simulink model "matrix"  (R2023a)
settings: Solver=VariableStepAuto  StartTime=0.0  StopTime=1  RelTol=1e-3
libraries: spsDiodeLib x8, spsIGBTLib x8, spsVoltageMeasurementLib x2, spsACVoltageSourceLib x1, sps_lib x1, spsSeriesRLCBranchLib x1
settings Model: Creator=burra  LastModifiedBy=vande

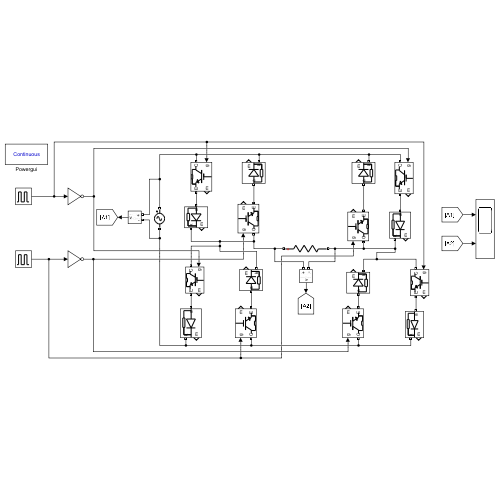
[thumbnail: Simulink's stored preview of the top-level diagram]
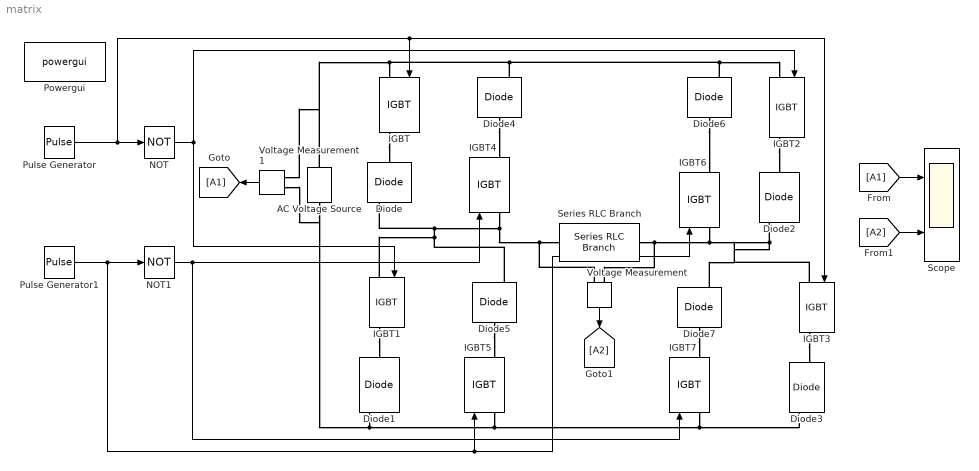
== system matrix ==
  AC Voltage Source : spsACVoltageSourceLib/AC Voltage Source  Amplitude=230  Phase=0  Frequency=50  SampleTime=0  Measurements=None  BusType=swing  Pref=10e3  Qref=0  Qmin=-inf  Qmax=+inf
  Diode{,1..7} (8 alike) : spsDiodeLib/Diode  Ron=0.001  Lon=0  Vf=0.8  IC=0  UseSnubber=0  Rs=500  Cs=250e-9  Measurements=on
  IGBT{,1..7} (8 alike) : spsIGBTLib/IGBT  Ron=0.001  Lon=0  Vf=1  Tf=1e-6  Tt=2e-6  IC=0  Rs=1e5  Cs=inf  Measurements=on
  NOT : Logic  Operator=NOT  IconShape=distinctive  AllPortsSameDT=off  OutDataTypeStr=boolean
  NOT1 : Logic  Operator=NOT  IconShape=distinctive  AllPortsSameDT=off  OutDataTypeStr=boolean
  Powergui : sps_lib/powergui  Priority=1  SimulationMode=Continuous  SampleTime=50e-6  frequency=60  Iterations=50  frequencyindice=50  Pbase=100e6  ErrMax=1e-4  UnitsV=kV  UnitsW=MW  buscounter=0  FunctionMessages=off  echomessages=off  EnableUseOfTLC=off  CurrentSourceSwitches=off  DisableSnubberDevices=off  DisableRonSwitches=off  DisableVfSwitches=off  DisplayEquations=off  AutomaticDiscreteSolvers=off  SolverType=Tustin/Backward Euler (TBE)  Interpol=off  ExternalGateDelay=off  methode=off  Ts=100  x0status=blocks  SPID=on  SwTol=0  HookPort=off  NonlinearTolerance=1e-4  nMaxIteration=100  ContinueOnMaxIteration=off  RestoreLinks=warning  ResistiveCurrentMeasurement=off  Frange=[0:2:500]  Ylog=off  Xlog=on  ShowGrid=off  save=off  variable=ZData  structure=0  ZoomFFT=off  StartTime=0.0  cycles=1  DisplayStyle=1  fundamental=60  FreqAxis=off  MaxFrequency=1000  frequencyindicesteady=1  RmsSteady=1  display=off
  Pulse Generator : DiscretePulseGenerator  PulseType=Time based  Period=0.001  PulseWidth=50
  Pulse Generator1 : DiscretePulseGenerator  PulseType=Time based  Period=0.001  PulseWidth=50
  Scope : Scope  NumInputPorts=2
  Series RLC Branch : spsSeriesRLCBranchLib/Series RLC Branch  LConnTagsString=__new0  RConnTagsString=__new0  BranchType=R  Resistance=1  Inductance=1e-3  SetiL0=off  InitialCurrent=0  Capacitance=1e-6  Setx0=off  InitialVoltage=0  Measurements=None
  Voltage Measurement : spsVoltageMeasurementLib/Voltage Measurement  PhasorSimulation=off  OutputType=Complex  PSBequivalent=0
  Voltage Measurement1 : spsVoltageMeasurementLib/Voltage Measurement  PhasorSimulation=off  OutputType=Complex  PSBequivalent=0
  wires:
  Pulse Generator/1 -> IGBT3/1, IGBT/1, NOT/1
  Pulse Generator1/1 -> IGBT6/1, IGBT5/1, NOT1/1
  NOT/1 -> IGBT2/1, IGBT1/1
  NOT1/1 -> IGBT4/1, IGBT7/1
  Voltage Measurement1/1 -> [A1]
  [A1] -> Scope/1
  [A2] -> Scope/2
  Voltage Measurement/1 -> [A2]
  connections:
  IGBT1/LConn1 -- Diode5/RConn1 -- Diode/RConn1 -- Voltage Measurement/LConn1 -- Series RLC Branch/LConn1 -- IGBT4/LConn1
  Diode6/RConn1 -- IGBT2/LConn1 -- Diode4/RConn1 -- Voltage Measurement1/LConn1 -- AC Voltage Source/RConn1 -- IGBT/LConn1
  Diode4/LConn1 -- IGBT4/RConn1
  IGBT/RConn1 -- Diode/LConn1
  IGBT2/RConn1 -- Diode2/LConn1
  Diode6/LConn1 -- IGBT6/RConn1
  Series RLC Branch/RConn1 -- Voltage Measurement/LConn2 -- IGBT3/LConn1 -- Diode7/RConn1 -- Diode2/RConn1 -- IGBT6/LConn1
  IGBT1/RConn1 -- Diode1/LConn1
  Diode5/LConn1 -- IGBT5/RConn1
  Diode1/RConn1 -- Voltage Measurement1/LConn2 -- AC Voltage Source/LConn1 -- IGBT5/LConn1 -- Diode3/RConn1 -- IGBT7/LConn1
  Diode7/LConn1 -- IGBT7/RConn1
  IGBT3/RConn1 -- Diode3/LConn1
